simulink model "Electrical_System_2018b_obfs"  (R2019b)
settings: Solver=VariableStepAuto  StartTime=0.0  StopTime=5  RelTol=1e-3  AbsTol=1e-3  EnableMultiTasking=on
InitFcn:
  | Steady_State_Initialisation;
StopFcn:
  | %sscexplore(simlog);
  | %Logging
undefined symbols (not defined in the file): abrlhklxvp, aexgmhuedq, afmfmjnutg, afpphrjpnc, ahuxbyvruc, alarvljztt, amxnyqmnuw, aodrlwvqie, aolhmuplyq, aqpmguuqkg, auesgwirzl, aurophlnng, awamelrhru, ayfhvxflxn, azxkacuhqc, babszerikg, bawhdqanwq, bevoqecvei, bltjvqbchx, bmqsuewujl, bsmyqjfgnf, btvjbsmnve, bywgxqeadw, bziaduxaer, bzmcmdqocb, bzsvyvetat, ccsjnrbsih, cdvenygxwh, cedkrnslhx, cjheorclzs, cjrdshrtqx, ckhavyhcza, ckxewznhlz, cmrcgyiplk, conenicnws, cqkejbgjnn, csfnuwymhe, cunupkhwbh, cwzfvzuxxh, dcadmadufn, dcfponivnv, ddtrqjrhjn, dfhoxvkqas, dfrhtcwpne, dfvomcagjv, djijwylxea, dnmeqksrrm, dnzewbdkaa, dsqcykyxav, dtswwlttmm, ecumpidjtv, edegaywrct, ejjjsmnejc, eknqnehjdz, emvdetzouf, esxbqkbahr, etnkkbreiq, eunoiiiirw, ewewcuedir, fatkfxdhtc ... (+386)
libraries: fl_lib x802, ee_lib x362, fl_ps_legacy_lib x160, nesl_utility x85
(part 16 of 26)

== system Electrical_System_2018b_obfs/Redacted_1221/Redacted_7996/Redacted_2/Redacted_38/Redacted_8107/Redacted_7529 ==
  Redacted_1084 : ee_lib/Semiconductors & Converters/Diode  ModelType=izdobyzqle  Vf=evihkhstbw V  Ron=vuuzcskhxp Ohm  Goff=mlnvudefzh S  prmExp=lejtfyvyux  I12=tabfzyvjjw A  V12=fmhjbmpmqb V  IS=owmyvxeefr A  ec=svhshwyrgx  I1=ljwwgiysfr A  V1=cxpndjgyrh V  RS=xmnymghsco Ohm  Tmeas=zghhcluqyd degC  N_series=cpqweisfkm  N_parallel=lexvmnvtgk  Rz=qmwaibykde Ohm  BV=drbkvafvno V  C_param=xxddurxsbn  CJ=xdxqdbopkt pF  CJ0=kptwwgjzso pF  VJ=hkmlapdavl V  Mgrad=vyzsmtybaj  Vvec=idvcnbeqxi V  Cvec=lhhotedrtn pF  FC=bewrjixdsy  Q_param=ivgezzsvid  iRM=kttgtaurdl A  iF=feyuhnjntw A  didt=wzaronjtgo A/us  trr_factor=xjeyfathbr  trr=gmgemqpikq ns  Qrr=psqfrowxwi s*uA  TT=klclxejlrf ns  tau=dytmmyuhbl ns  T_param=gahisfowsc  IS_T2=cvrsutiwlp A  I1_T2=lhcryknhzp A  V1_T2=nabkspnaxp V  Tmeas2=yxgzayqlzi degC  EG_param=qwryskkgkm  EG=oxgfzaipim eV  XTI_param=bjoagcqjsw  XTI=ycmlwmcwwf  dBVdT=dotvxllash V/K  Tdevice=ezkzuymnag degC  i_specify=off  i_priority=None  i=daydkonpxs A  i_nominal_specify=off  i_nominal_unit=A  i_nominal_value=blmtdukctw  v_specify=off  v_priority=None  v=akgpvqsdrg V  v_nominal_specify=off  v_nominal_unit=V  v_nominal_value=lygvltjuxz  i_capacitor_specify=off  i_capacitor_priority=None  i_capacitor=btazvuzoqw A  i_capacitor_nominal_specify=off  i_capacitor_nominal_unit=A  i_capacitor_nominal_value=mpfscvienm  v_capacitor_specify=off  v_capacitor_priority=None  v_capacitor=fmmkhztbpm V  v_capacitor_nominal_specify=off  v_capacitor_nominal_unit=V  v_capacitor_nominal_value=ltvznzjvwn  power_dissipated_specify=off  power_dissipated_priority=None  power_dissipated=jxwbertlfp W  power_dissipated_nominal_specify=off  power_dissipated_nominal_unit=W  power_dissipated_nominal_value=qtoemtvmie  thermal_network_parameterization=vtcsjudzim  Rth=heeowetwuv K/W  Rth_Foster=ruqyjqugrl K/W  thermal_mass_parameterization=envbmlquin  thermal_mass=kwknucpqzf J/K  thermal_mass_Foster=cqdqbkuljl J/K  thermal_time_constant=ngzwrugeai s  thermal_time_constant_Foster=bpqkuoqgpu s  thermal_mass_initial_temperatures=rhqgsoeffv degC
      settings: SourceProductName=Simscape Electrical  InternalSimscapePortConfiguration="{\"Bottom\":[],\"Left\":[{\"id\":\"p\",\"label\":\"\",\"type\":\"foundation.electrical.electrical\"},{\"id\":\"H\",\"label\":\"H\",\"type\":\"foundation.thermal.thermal\"}],\"Right\":[{\"id\":\"n\",\"label\":\"\",\"type\":\"foundation.electrical.electrical\"}],\"Top\":[]}"
  Redacted_1116 : ee_lib/Semiconductors & Converters/Diode  ModelType=fezxkqjgqt  Vf=fxigmtorpi V  Ron=gczbijkgdb Ohm  Goff=eezdenrgyt S  prmExp=mooftzwsze  I12=hrjfyjjrls A  V12=rpjtpkqqat V  IS=wddelpkxcd A  ec=wnwrwrhrqv  I1=lxjmeqhfps A  V1=hwunywjuky V  RS=qeymtoopbm Ohm  Tmeas=moiijwwbbr degC  N_series=tpmlovrlqd  N_parallel=mfzinvasat  Rz=ovydxazbex Ohm  BV=pxxjbuwfqz V  C_param=qpcursofjw  CJ=xcjuvsuivt pF  CJ0=izhwoolfnz pF  VJ=vpiestyydi V  Mgrad=cktkfzulrn  Vvec=sciesnzgxa V  Cvec=ffirljqncp pF  FC=ggluskildl  Q_param=ivvyfxrgkf  iRM=vqdtwwvmky A  iF=pvrysfcrbt A  didt=aeuywekxid A/us  trr_factor=nqhyqwmkdj  trr=iqctnvzxva ns  Qrr=isykhlqcxv s*uA  TT=ebdjbikpxl ns  tau=braofdeijp ns  T_param=rwhudzydrl  IS_T2=ahyaxsqykv A  I1_T2=yqxbhliehb A  V1_T2=cahaepnczu V  Tmeas2=rcpxcpgkrc degC  EG_param=ajpcsxcgmn  EG=mkbrzouimp eV  XTI_param=fgrnhizmgq  XTI=rtivxbansn  dBVdT=bztvayfwko V/K  Tdevice=fwkbokttbz degC  i_specify=off  i_priority=None  i=frjerhxssh A  i_nominal_specify=off  i_nominal_unit=A  i_nominal_value=xtkoagasgf  v_specify=off  v_priority=None  v=ltequmallb V  v_nominal_specify=off  v_nominal_unit=V  v_nominal_value=nmmakwdacx  i_capacitor_specify=off  i_capacitor_priority=None  i_capacitor=oexcyamlgf A  i_capacitor_nominal_specify=off  i_capacitor_nominal_unit=A  i_capacitor_nominal_value=tsglkvwluo  v_capacitor_specify=off  v_capacitor_priority=None  v_capacitor=uttypvaate V  v_capacitor_nominal_specify=off  v_capacitor_nominal_unit=V  v_capacitor_nominal_value=rmuymllcxy  power_dissipated_specify=off  power_dissipated_priority=None  power_dissipated=pikztcggua W  power_dissipated_nominal_specify=off  power_dissipated_nominal_unit=W  power_dissipated_nominal_value=wdovbxesnv  thermal_network_parameterization=jzuiubyezr  Rth=zuswrtrzus K/W  Rth_Foster=mncqifigaw K/W  thermal_mass_parameterization=xdyzfyucfr  thermal_mass=digaqnegbt J/K  thermal_mass_Foster=rlibwejjxp J/K  thermal_time_constant=dtpvzfxfdr s  thermal_time_constant_Foster=lltkuepcfr s  thermal_mass_initial_temperatures=qrjsznixcz degC
      settings: SourceProductName=Simscape Electrical  InternalSimscapePortConfiguration="{\"Bottom\":[],\"Left\":[{\"id\":\"p\",\"label\":\"\",\"type\":\"foundation.electrical.electrical\"},{\"id\":\"H\",\"label\":\"H\",\"type\":\"foundation.thermal.thermal\"}],\"Right\":[{\"id\":\"n\",\"label\":\"\",\"type\":\"foundation.electrical.electrical\"}],\"Top\":[]}"
  Redacted_3535 : ee_lib/Passive/Thermal/Thermal Resistor  R=nnovauibfc K/W  T_specify=off  T_priority=None  T=smooypmoft K  T_nominal_specify=off  T_nominal_unit=K  T_nominal_value=kuntnrwjbm  Q_specify=off  Q_priority=None  Q=ffwudhgepl W  Q_nominal_specify=off  Q_nominal_unit=W  Q_nominal_value=dtpumxdoon
      settings: SourceProductName=Simscape Electrical  SourceProductBaseCode=PS  InternalSimscapePortConfiguration="{\"Bottom\":[],\"Left\":[{\"id\":\"A\",\"label\":\"A\",\"type\":\"foundation.thermal.thermal\"}],\"Right\":[{\"id\":\"B\",\"label\":\"B\",\"type\":\"foundation.thermal.thermal\"}],\"Top\":[]}"
  Redacted_4646 : fl_lib/Electrical/Electrical Elements/Switch  R_closed=pqgaemrczs Ohm  G_open=ijstyudrez 1/Ohm  Threshold=xtptocpmir  i_specify=off  i_priority=None  i=ciwbetxiqp A  i_nominal_specify=off  i_nominal_unit=A  i_nominal_value=enaqgcdnlz  v_specify=off  v_priority=None  v=vzxbmtbrih V  v_nominal_specify=off  v_nominal_unit=V  v_nominal_value=wsynujvvrc
      settings: SourceProductName=Simscape
  Redacted_5773 : ee_lib/Passive/Thermal/Thermal Resistor  R=edegaywrct K/W  T_specify=off  T_priority=None  T=ckxewznhlz K  T_nominal_specify=off  T_nominal_unit=K  T_nominal_value=gkohcrexhh  Q_specify=off  Q_priority=None  Q=ubkoftignu W  Q_nominal_specify=off  Q_nominal_unit=W  Q_nominal_value=dmlagltzis
      settings: SourceProductName=Simscape Electrical  SourceProductBaseCode=PS  InternalSimscapePortConfiguration="{\"Bottom\":[],\"Left\":[{\"id\":\"A\",\"label\":\"A\",\"type\":\"foundation.thermal.thermal\"}],\"Right\":[{\"id\":\"B\",\"label\":\"B\",\"type\":\"foundation.thermal.thermal\"}],\"Top\":[]}"
  Redacted_6378 : fl_lib/Electrical/Electrical Elements/Switch  R_closed=whblxebmyo Ohm  G_open=pswlapjyse 1/Ohm  Threshold=pwweavvhgn  i_specify=off  i_priority=None  i=elbzoqtfyk A  i_nominal_specify=off  i_nominal_unit=A  i_nominal_value=sbenumnblt  v_specify=off  v_priority=None  v=vclonruutc V  v_nominal_specify=off  v_nominal_unit=V  v_nominal_value=xzmfluzccj
      settings: SourceProductName=Simscape
  Redacted_6493 : ee_lib/Semiconductors & Converters/Diode  ModelType=vttiaricbl  Vf=ogmshccous V  Ron=clhmvbtmpj Ohm  Goff=qlartobjid S  prmExp=yehkiyfwrf  I12=uxupgfdefd A  V12=fnuyckqxoq V  IS=gijoawrwfl A  ec=jacbxiiccp  I1=fgncvolvfb A  V1=onmmvewocq V  RS=otizmpmqay Ohm  Tmeas=kapmscogpw degC  N_series=qithjwaybs  N_parallel=gzsiinkylg  Rz=mycurxzcbk Ohm  BV=rewmblcdnc V  C_param=whbhsgwygj  CJ=vcfjucyupa pF  CJ0=xlhglqasyv pF  VJ=qosroxbxnj V  Mgrad=hkxiwvlmct  Vvec=oruqsfqddv V  Cvec=sashthzyhc pF  FC=xhlcguewdu  Q_param=ixrezpchhb  iRM=djiqriviqu A  iF=hegkfqrgrh A  didt=xbnqhutjlk A/us  trr_factor=dzlursyiar  trr=ecuaptzqel ns  Qrr=imqebfbhyx s*uA  TT=dymphevecl ns  tau=sblfgxlvjk ns  T_param=xyqfplnupv  IS_T2=uxlhlnzgja A  I1_T2=cyfpvxxmef A  V1_T2=dbwddhswgd V  Tmeas2=zlvkqtpnfx degC  EG_param=fcgsavfugx  EG=jbtqkskxko eV  XTI_param=buvkrschfc  XTI=qctkrmjsmi  dBVdT=kyilrmqoag V/K  Tdevice=tvzbjueohw degC  i_specify=off  i_priority=None  i=wgxzavfjwv A  i_nominal_specify=off  i_nominal_unit=A  i_nominal_value=zeyksugkif  v_specify=off  v_priority=None  v=knzxvrfofm V  v_nominal_specify=off  v_nominal_unit=V  v_nominal_value=chjlmmweiu  i_capacitor_specify=off  i_capacitor_priority=None  i_capacitor=mednscufnd A  i_capacitor_nominal_specify=off  i_capacitor_nominal_unit=A  i_capacitor_nominal_value=leufklsnbm  v_capacitor_specify=off  v_capacitor_priority=None  v_capacitor=xrcvmsmjec V  v_capacitor_nominal_specify=off  v_capacitor_nominal_unit=V  v_capacitor_nominal_value=tbidastozp  power_dissipated_specify=off  power_dissipated_priority=None  power_dissipated=hpegcrwzwe W  power_dissipated_nominal_specify=off  power_dissipated_nominal_unit=W  power_dissipated_nominal_value=ueblnqxpvf  thermal_network_parameterization=hkgyvucefr  Rth=bprjyiudmm K/W  Rth_Foster=bqwxkgbgel K/W  thermal_mass_parameterization=gnzfaualyz  thermal_mass=qgoqgvzmhv J/K  thermal_mass_Foster=lrajjjlskm J/K  thermal_time_constant=ffhhmbgnyr s  thermal_time_constant_Foster=dwjhaccnar s  thermal_mass_initial_temperatures=clzednejpb degC
      settings: SourceProductName=Simscape Electrical  InternalSimscapePortConfiguration="{\"Bottom\":[],\"Left\":[{\"id\":\"p\",\"label\":\"\",\"type\":\"foundation.electrical.electrical\"},{\"id\":\"H\",\"label\":\"H\",\"type\":\"foundation.thermal.thermal\"}],\"Right\":[{\"id\":\"n\",\"label\":\"\",\"type\":\"foundation.electrical.electrical\"}],\"Top\":[]}"
  Redacted_6995 : ee_lib/Semiconductors & Converters/Diode  ModelType=jutammamgf  Vf=phixztrybu V  Ron=wnueokvcjp Ohm  Goff=tlbagzjnli S  prmExp=qepetuupwd  I12=pipfumlpkp A  V12=cvdomcruuy V  IS=caphgfqgul A  ec=bfsyyglqre  I1=chsqwrduxs A  V1=pnvjrtaaxm V  RS=lnonjcbaes Ohm  Tmeas=uqgbdgyiqe degC  N_series=wzcnpegdoc  N_parallel=vzpnmjfana  Rz=jvagvrqcvr Ohm  BV=iowbeuhkbn V  C_param=zuyiiufywv  CJ=iafdabsqml pF  CJ0=krrwskzkzk pF  VJ=hcozynotnd V  Mgrad=qgebppotct  Vvec=rsjrazbslf V  Cvec=tqthplanse pF  FC=ggxesrxcvy  Q_param=npdtukbqqy  iRM=baufngyjqn A  iF=eaqdcbooap A  didt=zpmwgjwvhg A/us  trr_factor=lxzhpepuka  trr=lxionuhlzp ns  Qrr=cedutijpwi s*uA  TT=unwcmeqxzu ns  tau=bqcttgeatr ns  T_param=hnuznnjugk  IS_T2=heqzetlzuz A  I1_T2=zuzqagssvf A  V1_T2=jebzqvibaa V  Tmeas2=liqnbtkzkz degC  EG_param=paovebrsxo  EG=afafawlgir eV  XTI_param=eznhhwiwyq  XTI=pnvwrinkhd  dBVdT=ncvzhuvhdd V/K  Tdevice=xjszywknrp degC  i_specify=off  i_priority=None  i=ksmvescqii A  i_nominal_specify=off  i_nominal_unit=A  i_nominal_value=vdbtoezmns  v_specify=off  v_priority=None  v=mjrlqidlhj V  v_nominal_specify=off  v_nominal_unit=V  v_nominal_value=kpyhvjeelx  i_capacitor_specify=off  i_capacitor_priority=None  i_capacitor=rleowstiyj A  i_capacitor_nominal_specify=off  i_capacitor_nominal_unit=A  i_capacitor_nominal_value=cqjcqxpbep  v_capacitor_specify=off  v_capacitor_priority=None  v_capacitor=atjaslazmh V  v_capacitor_nominal_specify=off  v_capacitor_nominal_unit=V  v_capacitor_nominal_value=wpxewlzklj  power_dissipated_specify=off  power_dissipated_priority=None  power_dissipated=mwdylpnyws W  power_dissipated_nominal_specify=off  power_dissipated_nominal_unit=W  power_dissipated_nominal_value=jrnlbozeni  thermal_network_parameterization=dbphpnpgiy  Rth=xxmcnnlxls K/W  Rth_Foster=owybowsyqi K/W  thermal_mass_parameterization=fipqtfbsom  thermal_mass=sufocoiqer J/K  thermal_mass_Foster=kpdllifdhl J/K  thermal_time_constant=miladgbser s  thermal_time_constant_Foster=ttjplmfpfh s  thermal_mass_initial_temperatures=yzetsrudhm degC
      settings: SourceProductName=Simscape Electrical  InternalSimscapePortConfiguration="{\"Bottom\":[],\"Left\":[{\"id\":\"p\",\"label\":\"\",\"type\":\"foundation.electrical.electrical\"},{\"id\":\"H\",\"label\":\"H\",\"type\":\"foundation.thermal.thermal\"}],\"Right\":[{\"id\":\"n\",\"label\":\"\",\"type\":\"foundation.electrical.electrical\"}],\"Top\":[]}"
  Redacted_7501 : fl_lib/Electrical/Electrical Elements/Switch  R_closed=hkpufaysry Ohm  G_open=gpzouyuqvs 1/Ohm  Threshold=qzaeawbkdg  i_specify=off  i_priority=None  i=gtsknxhqqy A  i_nominal_specify=off  i_nominal_unit=A  i_nominal_value=zlbtgeochj  v_specify=off  v_priority=None  v=dywgqxyfrf V  v_nominal_specify=off  v_nominal_unit=V  v_nominal_value=tmhxabklck
      settings: SourceProductName=Simscape
  Redacted_7912 : ee_lib/Semiconductors & Converters/Diode  ModelType=rwagzwdqyn  Vf=iprlzxekyz V  Ron=ezbutranua Ohm  Goff=dhqmfjsjtj S  prmExp=cuexlqtxbd  I12=huvborskst A  V12=yjowgrbbok V  IS=recqqdaika A  ec=maqoiaeowd  I1=dfgsziufhg A  V1=jfgkxmlxal V  RS=rwxzegglbh Ohm  Tmeas=jioffbrnci degC  N_series=fvxphqozbm  N_parallel=klvniviixg  Rz=lchiewuqih Ohm  BV=jvermwbkfz V  C_param=aeaujmzfqy  CJ=rqoxxznype pF  CJ0=fgmgeudhfq pF  VJ=dirbounqek V  Mgrad=rzoyersdzn  Vvec=uohghsdlzr V  Cvec=sbaqfspfgh pF  FC=nnbelozaaf  Q_param=otgxpunumz  iRM=nvsewfidxu A  iF=stbhkngzcy A  didt=qcdzydoljm A/us  trr_factor=finkzecfng  trr=obgbvrcfxj ns  Qrr=hjehgagare s*uA  TT=fxfsjglodu ns  tau=lgetnnmyzx ns  T_param=mpmzudimoq  IS_T2=ixsjntuwes A  I1_T2=nlkfhnvcta A  V1_T2=ihjdtzpuop V  Tmeas2=tlrwraxkbp degC  EG_param=xxzzjsgowy  EG=osmqxpygwj eV  XTI_param=xnphfrlzyj  XTI=lyfutvjcve  dBVdT=zpjxgnsdoi V/K  Tdevice=ejwhigvruq degC  i_specify=off  i_priority=None  i=fjexkzazrq A  i_nominal_specify=off  i_nominal_unit=A  i_nominal_value=fuktovoelv  v_specify=off  v_priority=None  v=wqxfyskvyj V  v_nominal_specify=off  v_nominal_unit=V  v_nominal_value=kqzybxpjnu  i_capacitor_specify=off  i_capacitor_priority=None  i_capacitor=ofanbrxoer A  i_capacitor_nominal_specify=off  i_capacitor_nominal_unit=A  i_capacitor_nominal_value=joivzqgqdu  v_capacitor_specify=off  v_capacitor_priority=None  v_capacitor=slkzwjrqcn V  v_capacitor_nominal_specify=off  v_capacitor_nominal_unit=V  v_capacitor_nominal_value=btklwtqjaq  power_dissipated_specify=off  power_dissipated_priority=None  power_dissipated=bkyjzqujvp W  power_dissipated_nominal_specify=off  power_dissipated_nominal_unit=W  power_dissipated_nominal_value=wvaevrhbzy  thermal_network_parameterization=ntnnypyupt  Rth=fjtewgrqlr K/W  Rth_Foster=rcjajmoogt K/W  thermal_mass_parameterization=wipcxjewms  thermal_mass=ljwuxclnun J/K  thermal_mass_Foster=llxyimdsaa J/K  thermal_time_constant=dxqpwebpua s  thermal_time_constant_Foster=pglxwtomtd s  thermal_mass_initial_temperatures=hidbrzofoy degC
      settings: SourceProductName=Simscape Electrical  InternalSimscapePortConfiguration="{\"Bottom\":[],\"Left\":[{\"id\":\"p\",\"label\":\"\",\"type\":\"foundation.electrical.electrical\"},{\"id\":\"H\",\"label\":\"H\",\"type\":\"foundation.thermal.thermal\"}],\"Right\":[{\"id\":\"n\",\"label\":\"\",\"type\":\"foundation.electrical.electrical\"}],\"Top\":[]}"
  Redacted_8948 : ee_lib/Semiconductors & Converters/Diode  ModelType=zkbpdzndof  Vf=kzhddisigf V  Ron=dwbhxmmusu Ohm  Goff=bovrirpbke S  prmExp=ivxatfylqk  I12=zvwbuodsjc A  V12=hygnuemoix V  IS=tfwnmkcsyy A  ec=zckyboqwbh  I1=gvubnhdebg A  V1=kunekwhnwv V  RS=ecflormmke Ohm  Tmeas=gtkqfbhchd degC  N_series=zexkrzwhec  N_parallel=wsgrspekur  Rz=shpvzfgjkm Ohm  BV=ccrgfqifiu V  C_param=jqwkikvznj  CJ=pnytyzyvdj pF  CJ0=lnkqhrgppk pF  VJ=uipwhuhyam V  Mgrad=iufkrvrvhb  Vvec=xkhpmfjhdd V  Cvec=uybicdtekz pF  FC=fimwjtluum  Q_param=ctngtcsbuv  iRM=irhzfxednb A  iF=qottmbjvjb A  didt=eltqzqpenk A/us  trr_factor=vqicmosdaw  trr=wqdiphslkd ns  Qrr=xasjjvxkjf s*uA  TT=lfeufmusqp ns  tau=blqvezoiur ns  T_param=okzhatcrhj  IS_T2=cdpladztvs A  I1_T2=cfzfnsrxin A  V1_T2=isvyuxqhap V  Tmeas2=uhkmdahdaa degC  EG_param=hrwywwihcq  EG=euxrsrmpjb eV  XTI_param=yykzdnakfo  XTI=zqzfakywur  dBVdT=yajojhgtsn V/K  Tdevice=hzqpbccwul degC  i_specify=off  i_priority=None  i=nyprrbxiwt A  i_nominal_specify=off  i_nominal_unit=A  i_nominal_value=qchgoadyeu  v_specify=off  v_priority=None  v=cxjaxlbuuh V  v_nominal_specify=off  v_nominal_unit=V  v_nominal_value=enugljpiad  i_capacitor_specify=off  i_capacitor_priority=None  i_capacitor=fyumucjymc A  i_capacitor_nominal_specify=off  i_capacitor_nominal_unit=A  i_capacitor_nominal_value=mwslhozglg  v_capacitor_specify=off  v_capacitor_priority=None  v_capacitor=hatozsragm V  v_capacitor_nominal_specify=off  v_capacitor_nominal_unit=V  v_capacitor_nominal_value=nedivgajsa  power_dissipated_specify=off  power_dissipated_priority=None  power_dissipated=dxpmizpfad W  power_dissipated_nominal_specify=off  power_dissipated_nominal_unit=W  power_dissipated_nominal_value=mfhacyeutq  thermal_network_parameterization=kkiafvbnuz  Rth=dhbknzzzyf K/W  Rth_Foster=krirsjbigm K/W  thermal_mass_parameterization=ncxhbuwddl  thermal_mass=ixwloffvbv J/K  thermal_mass_Foster=ysigxentbo J/K  thermal_time_constant=xcztavzciz s  thermal_time_constant_Foster=ysamghlcvt s  thermal_mass_initial_temperatures=bozfzmyjvc degC
      settings: SourceProductName=Simscape Electrical  InternalSimscapePortConfiguration="{\"Bottom\":[],\"Left\":[{\"id\":\"p\",\"label\":\"\",\"type\":\"foundation.electrical.electrical\"},{\"id\":\"H\",\"label\":\"H\",\"type\":\"foundation.thermal.thermal\"}],\"Right\":[{\"id\":\"n\",\"label\":\"\",\"type\":\"foundation.electrical.electrical\"}],\"Top\":[]}"
  Redacted_9145 : ee_lib/Passive/Thermal/Thermal Resistor  R=ayfhvxflxn K/W  T_specify=off  T_priority=None  T=tjccnrtnkd K  T_nominal_specify=off  T_nominal_unit=K  T_nominal_value=fepcbhdcxp  Q_specify=off  Q_priority=None  Q=yjxepqleci W  Q_nominal_specify=off  Q_nominal_unit=W  Q_nominal_value=ednxibyxiq
      settings: SourceProductName=Simscape Electrical  SourceProductBaseCode=PS  InternalSimscapePortConfiguration="{\"Bottom\":[],\"Left\":[{\"id\":\"A\",\"label\":\"A\",\"type\":\"foundation.thermal.thermal\"}],\"Right\":[{\"id\":\"B\",\"label\":\"B\",\"type\":\"foundation.thermal.thermal\"}],\"Top\":[]}"
  Redacted_9512 : ee_lib/Passive/Thermal/Thermal Resistor  R=qdhdwuufms K/W  T_specify=off  T_priority=None  T=qpsjblfwaq K  T_nominal_specify=off  T_nominal_unit=K  T_nominal_value=jijbdnsmls  Q_specify=off  Q_priority=None  Q=isaanbfiuu W  Q_nominal_specify=off  Q_nominal_unit=W  Q_nominal_value=pquhzcjzlx
      settings: SourceProductName=Simscape Electrical  SourceProductBaseCode=PS  InternalSimscapePortConfiguration="{\"Bottom\":[],\"Left\":[{\"id\":\"A\",\"label\":\"A\",\"type\":\"foundation.thermal.thermal\"}],\"Right\":[{\"id\":\"B\",\"label\":\"B\",\"type\":\"foundation.thermal.thermal\"}],\"Top\":[]}"
  Redacted_3998 : PMIOPort  Side=Left
  Redacted_3025 : PMIOPort  Port=2  Side=Left
  Redacted_376 : PMIOPort  Port=3  Side=Left
  Redacted_4990 : PMIOPort  Port=4  Side=Right
  Redacted_668 : PMIOPort  Port=5  Side=Right
  Redacted_6324 : PMIOPort  Port=6  Side=Right
  Redacted_5539 : PMIOPort  Port=7  Side=Left
  Redacted_7776 : PMIOPort  Port=8  Side=Right
  connections:
  Redacted_6493/LConn1 -- Redacted_3025/RConn1 -- Redacted_1116/RConn1
  Redacted_6493/RConn1 -- Redacted_4646/LConn1 -- Redacted_1116/LConn1
  Redacted_5773/LConn1 -- Redacted_8948/LConn2 -- Redacted_1084/LConn2
  Redacted_4990/RConn1 -- Redacted_6378/RConn2
  Redacted_1084/LConn1 -- Redacted_6378/LConn1 -- Redacted_8948/RConn1
  Redacted_8948/LConn1 -- Redacted_3998/RConn1 -- Redacted_1084/RConn1
  Redacted_9145/RConn1 -- Redacted_3535/RConn1 -- Redacted_9512/LConn1 -- Redacted_5773/RConn1
  Redacted_7912/LConn1 -- Redacted_376/RConn1 -- Redacted_6995/RConn1
  Redacted_6324/RConn1 -- Redacted_7501/RConn2
  Redacted_7776/RConn1 -- Redacted_7501/RConn1 -- Redacted_4646/RConn1 -- Redacted_6378/RConn1
  Redacted_668/RConn1 -- Redacted_4646/RConn2
  Redacted_6995/LConn1 -- Redacted_7501/LConn1 -- Redacted_7912/RConn1
  Redacted_6995/LConn2 -- Redacted_3535/LConn1 -- Redacted_7912/LConn2
  Redacted_9512/RConn1 -- Redacted_5539/RConn1
  Redacted_6493/LConn2 -- Redacted_1116/LConn2 -- Redacted_9145/LConn1

== system Electrical_System_2018b_obfs/Redacted_1221/Redacted_7996/Redacted_2/Redacted_38/Redacted_8107/Redacted_8444 ==
  Neutral_Negative : Subsystem  VariantControl=Variant1
  Positive_Neutral : Subsystem  VariantControl=Variant3
  Redacted_3917 : Subsystem  VariantControl=Variant2
  Redacted_8974 : PMIOPort  Side=Left
  Redacted_9727 : PMIOPort  Port=2  Side=Left
  Redacted_5818 : PMIOPort  Port=3  Side=Left
  Redacted_9930 : PMIOPort  Port=4  Side=Right
  Redacted_8840 : PMIOPort  Port=5  Side=Right

== system Electrical_System_2018b_obfs/Redacted_1221/Redacted_7996/Redacted_7418/Redacted_4377/Redacted_6082/Redacted_1335 ==
  Redacted_1591 : ee_lib/Semiconductors & Converters/Diode  ModelType=eepsypmlnm  Vf=vsdkpxkdvt V  Ron=hvipwyltcs Ohm  Goff=pncgtdpcky S  prmExp=ywnmgnebdg  I12=pijcksfllq A  V12=sokkewuwnq V  IS=lenjbmkbmu A  ec=usrydsfczj  I1=diflzejvue A  V1=ondqlqjixt V  RS=mmlszzuage Ohm  Tmeas=npymjxtxff degC  N_series=uwgycohtvj  N_parallel=vvktvyaksv  Rz=csndwjwvcs Ohm  BV=siuhniwsas V  C_param=mqmeyzacus  CJ=pspkjiflhw pF  CJ0=mkzhvuscrv pF  VJ=cxyxmemllb V  Mgrad=kwjdstgiqi  Vvec=rfkmbedwbl V  Cvec=tzcpccccyr pF  FC=tzhyramxnn  Q_param=jtaiadwcvb  iRM=teewqjimfa A  iF=dkuaowzmzk A  didt=wswqfekgti A/us  trr_factor=vgbmpjncqd  trr=qytitrwxvl ns  Qrr=jukjiwceed s*uA  TT=vfhkswzpii ns  tau=bcxefnpqla ns  T_param=knzoykoruc  IS_T2=wmrtfwgfyn A  I1_T2=wwatewxxmj A  V1_T2=vcmdipevcj V  Tmeas2=slejovgnym degC  EG_param=yrmdwgjpga  EG=obqdoxighd eV  XTI_param=hiiulsmtnp  XTI=fzvxbjgrlx  dBVdT=tcetjpxzuo V/K  Tdevice=jhymtvpuuv degC  i_specify=off  i_priority=None  i=lxkrvrufkt A  i_nominal_specify=off  i_nominal_unit=A  i_nominal_value=fptpkrapsh  v_specify=off  v_priority=None  v=hnwpggrdrb V  v_nominal_specify=off  v_nominal_unit=V  v_nominal_value=loyliznani  i_capacitor_specify=off  i_capacitor_priority=None  i_capacitor=qntetqcfew A  i_capacitor_nominal_specify=off  i_capacitor_nominal_unit=A  i_capacitor_nominal_value=bhetqfpmna  v_capacitor_specify=off  v_capacitor_priority=None  v_capacitor=qmuuchuxyz V  v_capacitor_nominal_specify=off  v_capacitor_nominal_unit=V  v_capacitor_nominal_value=vvvpkitexs  power_dissipated_specify=off  power_dissipated_priority=None  power_dissipated=kbjvtlpgfd W  power_dissipated_nominal_specify=off  power_dissipated_nominal_unit=W  power_dissipated_nominal_value=jvdnwocntn  thermal_network_parameterization=yoawbybtkl  Rth=uknyprueob K/W  Rth_Foster=quhjgsiudl K/W  thermal_mass_parameterization=atrvywscev  thermal_mass=gtmjoozywy J/K  thermal_mass_Foster=hdtqidrsds J/K  thermal_time_constant=adrtjfdoqm s  thermal_time_constant_Foster=lcosfsblai s  thermal_mass_initial_temperatures=kqftjagahg degC
      settings: SourceProductName=Simscape Electrical  InternalSimscapePortConfiguration="{\"Bottom\":[],\"Left\":[{\"id\":\"p\",\"label\":\"\",\"type\":\"foundation.electrical.electrical\"},{\"id\":\"H\",\"label\":\"H\",\"type\":\"foundation.thermal.thermal\"}],\"Right\":[{\"id\":\"n\",\"label\":\"\",\"type\":\"foundation.electrical.electrical\"}],\"Top\":[]}"
  Redacted_1669 : ee_lib/Passive/Thermal/Thermal Resistor  R=ejjjsmnejc K/W  T_specify=off  T_priority=None  T=mbytgkvqdk K  T_nominal_specify=off  T_nominal_unit=K  T_nominal_value=uvrqbhbcsu  Q_specify=off  Q_priority=None  Q=fryoumgfor W  Q_nominal_specify=off  Q_nominal_unit=W  Q_nominal_value=qudqfymccr
      settings: SourceProductName=Simscape Electrical  SourceProductBaseCode=PS  InternalSimscapePortConfiguration="{\"Bottom\":[],\"Left\":[{\"id\":\"A\",\"label\":\"A\",\"type\":\"foundation.thermal.thermal\"}],\"Right\":[{\"id\":\"B\",\"label\":\"B\",\"type\":\"foundation.thermal.thermal\"}],\"Top\":[]}"
  Redacted_4093 : fl_lib/Electrical/Electrical Elements/Switch  R_closed=bbadzxwyew Ohm  G_open=fzmtkxgwpd 1/Ohm  Threshold=dfvomcagjv  i_specify=off  i_priority=None  i=ohbeugqvip A  i_nominal_specify=off  i_nominal_unit=A  i_nominal_value=exxqjlbakz  v_specify=off  v_priority=None  v=rdiaxwucpj V  v_nominal_specify=off  v_nominal_unit=V  v_nominal_value=azkctcjsnz
      settings: SourceProductName=Simscape
  Redacted_5466 : ee_lib/Passive/Thermal/Thermal Resistor  R=wdtmondimm K/W  T_specify=off  T_priority=None  T=wrtafdzvbh K  T_nominal_specify=off  T_nominal_unit=K  T_nominal_value=fiihiabjan  Q_specify=off  Q_priority=None  Q=ypouestzei W  Q_nominal_specify=off  Q_nominal_unit=W  Q_nominal_value=mabqlhycjh
      settings: SourceProductName=Simscape Electrical  SourceProductBaseCode=PS  InternalSimscapePortConfiguration="{\"Bottom\":[],\"Left\":[{\"id\":\"A\",\"label\":\"A\",\"type\":\"foundation.thermal.thermal\"}],\"Right\":[{\"id\":\"B\",\"label\":\"B\",\"type\":\"foundation.thermal.thermal\"}],\"Top\":[]}"
  Redacted_7324 : fl_lib/Electrical/Electrical Elements/Switch  R_closed=omfvajnpfd Ohm  G_open=ipqnezpryn 1/Ohm  Threshold=mmcsavdyob  i_specify=off  i_priority=None  i=qwnjhvyruv A  i_nominal_specify=off  i_nominal_unit=A  i_nominal_value=zmauchnwye  v_specify=off  v_priority=None  v=ufnknxdamw V  v_nominal_specify=off  v_nominal_unit=V  v_nominal_value=edufhutzre
      settings: SourceProductName=Simscape
  Redacted_9050 : ee_lib/Passive/Thermal/Thermal Resistor  R=gnxjfqgycd K/W  T_specify=off  T_priority=None  T=dtswwlttmm K  T_nominal_specify=off  T_nominal_unit=K  T_nominal_value=iuxynuhpbk  Q_specify=off  Q_priority=None  Q=etqvxuddqu W  Q_nominal_specify=off  Q_nominal_unit=W  Q_nominal_value=jpdxcuslyz
      settings: SourceProductName=Simscape Electrical  SourceProductBaseCode=PS  InternalSimscapePortConfiguration="{\"Bottom\":[],\"Left\":[{\"id\":\"A\",\"label\":\"A\",\"type\":\"foundation.thermal.thermal\"}],\"Right\":[{\"id\":\"B\",\"label\":\"B\",\"type\":\"foundation.thermal.thermal\"}],\"Top\":[]}"
  Redacted_998 : ee_lib/Semiconductors & Converters/Diode  ModelType=jjfughauiv  Vf=eaqvjmxxyg V  Ron=canwxvkyyq Ohm  Goff=fylhafqfdf S  prmExp=dyvujabdmn  I12=kttaerjvea A  V12=kesibchmqe V  IS=cnmgoowrsx A  ec=wmgmtbxlpj  I1=kbcmpxrtrl A  V1=bxdgeigcbm V  RS=aqtkcecpuq Ohm  Tmeas=jagkxxxouu degC  N_series=eijeaxwsbs  N_parallel=gnezyptovg  Rz=ccfbjkqckh Ohm  BV=ibaqbmeitx V  C_param=qbielwnwyc  CJ=zriiuwgwxe pF  CJ0=dfescxdcew pF  VJ=cbwvhwuxfk V  Mgrad=imxnoqiriq  Vvec=scyvszjglj V  Cvec=fxqxkbblsd pF  FC=oefuhmbbrj  Q_param=azpytwrwfh  iRM=vffiognxml A  iF=obozmuzsag A  didt=gxjsoognzt A/us  trr_factor=ngilewgegt  trr=udeiywtgjk ns  Qrr=lseeyedphz s*uA  TT=rsgjgrebyr ns  tau=fnsxhspmvy ns  T_param=ompevgbwln  IS_T2=czoaxjmnms A  I1_T2=fomygjynsp A  V1_T2=axnvwvykbq V  Tmeas2=acusxjthih degC  EG_param=jvdcorncji  EG=cjbueeqdfy eV  XTI_param=ksyxmxcrgv  XTI=lqwkbkflhk  dBVdT=gzrvmvfdkg V/K  Tdevice=btlrowuowx degC  i_specify=off  i_priority=None  i=cbrwwtdksz A  i_nominal_specify=off  i_nominal_unit=A  i_nominal_value=tdaqsczgka  v_specify=off  v_priority=None  v=hzgsyifftd V  v_nominal_specify=off  v_nominal_unit=V  v_nominal_value=wwgtgaavtg  i_capacitor_specify=off  i_capacitor_priority=None  i_capacitor=ghdwybcfnr A  i_capacitor_nominal_specify=off  i_capacitor_nominal_unit=A  i_capacitor_nominal_value=patoccuvbb  v_capacitor_specify=off  v_capacitor_priority=None  v_capacitor=kipgljoorb V  v_capacitor_nominal_specify=off  v_capacitor_nominal_unit=V  v_capacitor_nominal_value=dyvrmzctdc  power_dissipated_specify=off  power_dissipated_priority=None  power_dissipated=ttfhebcktj W  power_dissipated_nominal_specify=off  power_dissipated_nominal_unit=W  power_dissipated_nominal_value=repcdnmkvu  thermal_network_parameterization=fmvbkiqdne  Rth=pazmfgafaa K/W  Rth_Foster=brspocefdd K/W  thermal_mass_parameterization=ykylewhfcq  thermal_mass=lrrjyxxvqd J/K  thermal_mass_Foster=vdbqyqwkrw J/K  thermal_time_constant=exusymqbix s  thermal_time_constant_Foster=asebieqyaj s  thermal_mass_initial_temperatures=hpkeovjooi degC
      settings: SourceProductName=Simscape Electrical  InternalSimscapePortConfiguration="{\"Bottom\":[],\"Left\":[{\"id\":\"p\",\"label\":\"\",\"type\":\"foundation.electrical.electrical\"},{\"id\":\"H\",\"label\":\"H\",\"type\":\"foundation.thermal.thermal\"}],\"Right\":[{\"id\":\"n\",\"label\":\"\",\"type\":\"foundation.electrical.electrical\"}],\"Top\":[]}"
  Redacted_3665 : PMIOPort  Side=Left
  Redacted_9500 : PMIOPort  Port=2  Side=Left
  Redacted_4916 : PMIOPort  Port=3  Side=Right
  Redacted_8865 : PMIOPort  Port=4  Side=Right
  Redacted_5813 : PMIOPort  Port=5  Side=Left
  Redacted_175 : PMIOPort  Port=6  Side=Right
  connections:
  Redacted_998/LConn2 -- Redacted_5466/LConn1
  Redacted_9050/RConn1 -- Redacted_5813/RConn1
  Redacted_8865/RConn1 -- Redacted_7324/RConn2
  Redacted_4093/RConn1 -- Redacted_7324/RConn1 -- Redacted_175/RConn1
  Redacted_1669/RConn1 -- Redacted_9050/LConn1 -- Redacted_5466/RConn1
  Redacted_3665/RConn1 -- Redacted_1591/RConn1
  Redacted_1591/LConn1 -- Redacted_4093/LConn1
  Redacted_4916/RConn1 -- Redacted_4093/RConn2
  Redacted_1591/LConn2 -- Redacted_1669/LConn1
  Redacted_998/RConn1 -- Redacted_7324/LConn1
  Redacted_998/LConn1 -- Redacted_9500/RConn1

== system Electrical_System_2018b_obfs/Redacted_1221/Redacted_7996/Redacted_7418/Redacted_4377/Redacted_6082/Redacted_1337 ==
  Redacted_1292 : ee_lib/Passive/Thermal/Thermal Resistor  R=gfxbaoqbci K/W  T_specify=off  T_priority=None  T=rvwtgoykrz K  T_nominal_specify=off  T_nominal_unit=K  T_nominal_value=dmbpfjxefx  Q_specify=off  Q_priority=None  Q=ozjvrxmttl W  Q_nominal_specify=off  Q_nominal_unit=W  Q_nominal_value=utwlydmrkv
      settings: SourceProductName=Simscape Electrical  SourceProductBaseCode=PS  InternalSimscapePortConfiguration="{\"Bottom\":[],\"Left\":[{\"id\":\"A\",\"label\":\"A\",\"type\":\"foundation.thermal.thermal\"}],\"Right\":[{\"id\":\"B\",\"label\":\"B\",\"type\":\"foundation.thermal.thermal\"}],\"Top\":[]}"
  Redacted_2743 : fl_lib/Electrical/Electrical Elements/Switch  R_closed=fsyfpyiukg Ohm  G_open=tvcalsacmg 1/Ohm  Threshold=ttjzchmxti  i_specify=off  i_priority=None  i=alduyvsbin A  i_nominal_specify=off  i_nominal_unit=A  i_nominal_value=loyuiwztoz  v_specify=off  v_priority=None  v=yjwvqchbme V  v_nominal_specify=off  v_nominal_unit=V  v_nominal_value=gjoornamne
      settings: SourceProductName=Simscape
  Redacted_3949 : ee_lib/Passive/Thermal/Thermal Resistor  R=mlcqaguecq K/W  T_specify=off  T_priority=None  T=hfikrglmxq K  T_nominal_specify=off  T_nominal_unit=K  T_nominal_value=dqcyvveaih  Q_specify=off  Q_priority=None  Q=qlchfeptuj W  Q_nominal_specify=off  Q_nominal_unit=W  Q_nominal_value=wfdtozcpan
      settings: SourceProductName=Simscape Electrical  SourceProductBaseCode=PS  InternalSimscapePortConfiguration="{\"Bottom\":[],\"Left\":[{\"id\":\"A\",\"label\":\"A\",\"type\":\"foundation.thermal.thermal\"}],\"Right\":[{\"id\":\"B\",\"label\":\"B\",\"type\":\"foundation.thermal.thermal\"}],\"Top\":[]}"
  Redacted_4700 : ee_lib/Passive/Thermal/Thermal Resistor  R=gvbddagohg K/W  T_specify=off  T_priority=None  T=qxaoehcsep K  T_nominal_specify=off  T_nominal_unit=K  T_nominal_value=nuvljcivmd  Q_specify=off  Q_priority=None  Q=cuqzitalwz W  Q_nominal_specify=off  Q_nominal_unit=W  Q_nominal_value=fpqwunqvoe
      settings: SourceProductName=Simscape Electrical  SourceProductBaseCode=PS  InternalSimscapePortConfiguration="{\"Bottom\":[],\"Left\":[{\"id\":\"A\",\"label\":\"A\",\"type\":\"foundation.thermal.thermal\"}],\"Right\":[{\"id\":\"B\",\"label\":\"B\",\"type\":\"foundation.thermal.thermal\"}],\"Top\":[]}"
  Redacted_6636 : fl_lib/Electrical/Electrical Elements/Switch  R_closed=cxbeobdwcz Ohm  G_open=vivqqcjshk 1/Ohm  Threshold=ihvrcphyhk  i_specify=off  i_priority=None  i=tlqvhosmyx A  i_nominal_specify=off  i_nominal_unit=A  i_nominal_value=zlqewbizhg  v_specify=off  v_priority=None  v=bylehoytgr V  v_nominal_specify=off  v_nominal_unit=V  v_nominal_value=nrfabisoae
      settings: SourceProductName=Simscape
  Redacted_7671 : ee_lib/Semiconductors & Converters/Diode  ModelType=olgpyqkyap  Vf=yiidzvusor V  Ron=onikhigqex Ohm  Goff=zwvbfgfjia S  prmExp=mbejlzmzoi  I12=iqvhxxtdcy A  V12=plenerjsyz V  IS=seajxixdni A  ec=smzaoqkpfi  I1=srlrouujzp A  V1=pbinkrtesx V  RS=maerkwpvvt Ohm  Tmeas=boxaemfztm degC  N_series=zwoiykegtu  N_parallel=jpsnlhanqe  Rz=rbegpmpdpq Ohm  BV=xqcgehksui V  C_param=smmkeyjtrn  CJ=mxoawofixc pF  CJ0=ucwkumcrgx pF  VJ=flpomdjhqn V  Mgrad=pogzifmwhx  Vvec=lvysrprkky V  Cvec=ofowmtrtdp pF  FC=xzrncupysx  Q_param=dpijdlsbtg  iRM=imlwlhdaoz A  iF=zahcqmmmsp A  didt=srqymkpvtu A/us  trr_factor=qutyflkerp  trr=alnpfsdzft ns  Qrr=pnoodsbkqz s*uA  TT=qzjfylnffu ns  tau=fiwiuyhrdw ns  T_param=wjqxjtpsrv  IS_T2=gnlmqposwz A  I1_T2=hhxkfrkipw A  V1_T2=otwkxldrvh V  Tmeas2=pqzzkcslrw degC  EG_param=rgdwepjzgz  EG=towtzjxupc eV  XTI_param=wnrxgiphjy  XTI=ifqnzmcann  dBVdT=izcgyclarw V/K  Tdevice=kuguckrfas degC  i_specify=off  i_priority=None  i=qwraxdsfza A  i_nominal_specify=off  i_nominal_unit=A  i_nominal_value=jrebnsmptq  v_specify=off  v_priority=None  v=faivdficoh V  v_nominal_specify=off  v_nominal_unit=V  v_nominal_value=bfbyoqyboc  i_capacitor_specify=off  i_capacitor_priority=None  i_capacitor=jrptblagdq A  i_capacitor_nominal_specify=off  i_capacitor_nominal_unit=A  i_capacitor_nominal_value=nibfyfosby  v_capacitor_specify=off  v_capacitor_priority=None  v_capacitor=whspnfsgdn V  v_capacitor_nominal_specify=off  v_capacitor_nominal_unit=V  v_capacitor_nominal_value=edempxzddr  power_dissipated_specify=off  power_dissipated_priority=None  power_dissipated=peqvvccveb W  power_dissipated_nominal_specify=off  power_dissipated_nominal_unit=W  power_dissipated_nominal_value=fvdlfslssq  thermal_network_parameterization=svzrqymosw  Rth=pzdrjrnlgr K/W  Rth_Foster=acztezytnk K/W  thermal_mass_parameterization=rgscyvsrgf  thermal_mass=kygdzlscru J/K  thermal_mass_Foster=dvwwklbogc J/K  thermal_time_constant=ykfmdcuqty s  thermal_time_constant_Foster=wgtknjdmmg s  thermal_mass_initial_temperatures=gjuzcynxks degC
      settings: SourceProductName=Simscape Electrical  InternalSimscapePortConfiguration="{\"Bottom\":[],\"Left\":[{\"id\":\"p\",\"label\":\"\",\"type\":\"foundation.electrical.electrical\"},{\"id\":\"H\",\"label\":\"H\",\"type\":\"foundation.thermal.thermal\"}],\"Right\":[{\"id\":\"n\",\"label\":\"\",\"type\":\"foundation.electrical.electrical\"}],\"Top\":[]}"
  Redacted_7804 : ee_lib/Semiconductors & Converters/Diode  ModelType=semwhebdsx  Vf=wlzsjodvxe V  Ron=kjejwwsved Ohm  Goff=idmqtjqxyt S  prmExp=ybznmgfoim  I12=ypbwuazhvu A  V12=kqbjrekczm V  IS=hvghirmuer A  ec=szvhwtedho  I1=dgebikxuyu A  V1=ekmofvolqe V  RS=jkmhfachtm Ohm  Tmeas=ahwyvfcpsr degC  N_series=atodrtceph  N_parallel=fkaurojkbb  Rz=egfgmfcnxn Ohm  BV=nluxtwjaqz V  C_param=qwanuoxlyf  CJ=ezbprdeztn pF  CJ0=peskbsrzop pF  VJ=vquvaidumd V  Mgrad=dfrmgpetae  Vvec=gunyxlsjla V  Cvec=nljyfkzkue pF  FC=itkqjjkjyc  Q_param=jgelcbblhx  iRM=jgdtjqhets A  iF=owsoaymscw A  didt=qmpgbmxkte A/us  trr_factor=hklhqkgxog  trr=veyznjjddh ns  Qrr=ejjniorttw s*uA  TT=suevkibuvy ns  tau=mawzmcgeyp ns  T_param=vqrqwbsxyj  IS_T2=ssgvnzergm A  I1_T2=kvtrmiebrl A  V1_T2=wfzbyspvvb V  Tmeas2=oidirsmqgk degC  EG_param=zfeizsafro  EG=pynrradmvc eV  XTI_param=chffuchcuy  XTI=acqdodawvu  dBVdT=ocrbmtpnpr V/K  Tdevice=zuabybkowd degC  i_specify=off  i_priority=None  i=bcjxinvzmi A  i_nominal_specify=off  i_nominal_unit=A  i_nominal_value=ackfofeggx  v_specify=off  v_priority=None  v=nodroimedg V  v_nominal_specify=off  v_nominal_unit=V  v_nominal_value=nhpkywzxmk  i_capacitor_specify=off  i_capacitor_priority=None  i_capacitor=gbqfpnudcs A  i_capacitor_nominal_specify=off  i_capacitor_nominal_unit=A  i_capacitor_nominal_value=jfrtogbkdj  v_capacitor_specify=off  v_capacitor_priority=None  v_capacitor=kykdbedtbj V  v_capacitor_nominal_specify=off  v_capacitor_nominal_unit=V  v_capacitor_nominal_value=bwzkdbziru  power_dissipated_specify=off  power_dissipated_priority=None  power_dissipated=crijfdzbch W  power_dissipated_nominal_specify=off  power_dissipated_nominal_unit=W  power_dissipated_nominal_value=gueeagjtzs  thermal_network_parameterization=nshhtosrtp  Rth=ymvhergmsa K/W  Rth_Foster=loktjbqqnk K/W  thermal_mass_parameterization=nxtgvvflim  thermal_mass=ipqsjmpyeh J/K  thermal_mass_Foster=pnnymgjcyt J/K  thermal_time_constant=fqlitfupll s  thermal_time_constant_Foster=ouoyijytio s  thermal_mass_initial_temperatures=hosplxrwnn degC
      settings: SourceProductName=Simscape Electrical  InternalSimscapePortConfiguration="{\"Bottom\":[],\"Left\":[{\"id\":\"p\",\"label\":\"\",\"type\":\"foundation.electrical.electrical\"},{\"id\":\"H\",\"label\":\"H\",\"type\":\"foundation.thermal.thermal\"}],\"Right\":[{\"id\":\"n\",\"label\":\"\",\"type\":\"foundation.electrical.electrical\"}],\"Top\":[]}"
  Redacted_9723 : PMIOPort  Side=Left
  Redacted_1721 : PMIOPort  Port=2  Side=Left
  Redacted_9002 : PMIOPort  Port=3  Side=Right
  Redacted_1469 : PMIOPort  Port=4  Side=Right
  Redacted_6509 : PMIOPort  Port=5  Side=Left
  Redacted_1134 : PMIOPort  Port=6  Side=Right
  connections:
  Redacted_7671/LConn2 -- Redacted_3949/LConn1
  Redacted_4700/RConn1 -- Redacted_6509/RConn1
  Redacted_1469/RConn1 -- Redacted_6636/RConn2
  Redacted_2743/RConn1 -- Redacted_6636/RConn1 -- Redacted_1134/RConn1
  Redacted_1292/RConn1 -- Redacted_4700/LConn1 -- Redacted_3949/RConn1
  Redacted_9723/RConn1 -- Redacted_7804/RConn1
  Redacted_7804/LConn1 -- Redacted_2743/LConn1
  Redacted_9002/RConn1 -- Redacted_2743/RConn2
  Redacted_7804/LConn2 -- Redacted_1292/LConn1
  Redacted_7671/RConn1 -- Redacted_6636/LConn1
  Redacted_7671/LConn1 -- Redacted_1721/RConn1

== system Electrical_System_2018b_obfs/Redacted_1221/Redacted_7996/Redacted_7418/Redacted_4377/Redacted_6082/Redacted_144 ==
  Neutral_Negative : Subsystem  VariantControl=Variant1
  Positive_Neutral : Subsystem  VariantControl=Variant3
  Redacted_9503 : Subsystem  VariantControl=Variant2
  Redacted_3879 : PMIOPort  Side=Left
  Redacted_3368 : PMIOPort  Port=2  Side=Left
  Redacted_9451 : PMIOPort  Port=3  Side=Left
  Redacted_8432 : PMIOPort  Port=4  Side=Right
  Redacted_6806 : PMIOPort  Port=5  Side=Right

== system Electrical_System_2018b_obfs/Redacted_1221/Redacted_7996/Redacted_7418/Redacted_4377/Redacted_6082/Redacted_1502 ==
  Redacted_179 : fl_lib/Electrical/Electrical Elements/Switch  R_closed=tpfczkzopb Ohm  G_open=guejjlojqy 1/Ohm  Threshold=qftxyxgxji  i_specify=off  i_priority=None  i=fngbtljzex A  i_nominal_specify=off  i_nominal_unit=A  i_nominal_value=pjpooffzff  v_specify=off  v_priority=None  v=bhcpirmmxz V  v_nominal_specify=off  v_nominal_unit=V  v_nominal_value=jucxroftek
      settings: SourceProductName=Simscape
  Redacted_1815 : ee_lib/Semiconductors & Converters/Diode  ModelType=dqnklwqfci  Vf=xjiqjpnnfi V  Ron=irekdgqkjv Ohm  Goff=iqhtpofome S  prmExp=knojfylagq  I12=bqxijupuhm A  V12=vzuzujtkpl V  IS=ydgywotbys A  ec=ayrfemqefn  I1=delsjshmli A  V1=dnxxzmtubb V  RS=wmjpjwroih Ohm  Tmeas=qmtcdggbzc degC  N_series=hklouwtkux  N_parallel=jrdkdmsmgo  Rz=tovmqbbrol Ohm  BV=avdgidxjam V  C_param=glqkxeqcta  CJ=chsawhndir pF  CJ0=ayexifqzkz pF  VJ=zqcsdkhphs V  Mgrad=fkespxnvnl  Vvec=dqwhbiesyc V  Cvec=niiqpqslou pF  FC=cwbzovuqpz  Q_param=ylelzifboz  iRM=omgsmfewsp A  iF=ichmjhkctu A  didt=orrasyxhrt A/us  trr_factor=zdlyciflht  trr=twfpakhxfd ns  Qrr=ipntneuszo s*uA  TT=mwhbnzgoop ns  tau=pfrrcdfsln ns  T_param=ytujlpikwb  IS_T2=jerhvoexxa A  I1_T2=jvyzqlfhuc A  V1_T2=zarbmnbtma V  Tmeas2=vwndrphzjd degC  EG_param=pcxlgqdkwd  EG=vtwlzbuxst eV  XTI_param=jcpfqvyxtb  XTI=phmgnxxjxe  dBVdT=orxkvsgthq V/K  Tdevice=oqbwtmobso degC  i_specify=off  i_priority=None  i=yajbkzqnsh A  i_nominal_specify=off  i_nominal_unit=A  i_nominal_value=iwrztftqvf  v_specify=off  v_priority=None  v=ewtusmxpho V  v_nominal_specify=off  v_nominal_unit=V  v_nominal_value=syahoyjouu  i_capacitor_specify=off  i_capacitor_priority=None  i_capacitor=vxlszklfgf A  i_capacitor_nominal_specify=off  i_capacitor_nominal_unit=A  i_capacitor_nominal_value=duzmsfhmfv  v_capacitor_specify=off  v_capacitor_priority=None  v_capacitor=grvkfvfijd V  v_capacitor_nominal_specify=off  v_capacitor_nominal_unit=V  v_capacitor_nominal_value=zqixbhndtz  power_dissipated_specify=off  power_dissipated_priority=None  power_dissipated=bveezoguoz W  power_dissipated_nominal_specify=off  power_dissipated_nominal_unit=W  power_dissipated_nominal_value=wuvllpdufa  thermal_network_parameterization=rsoaylhfgu  Rth=owtikceqjs K/W  Rth_Foster=lmkblyjvxa K/W  thermal_mass_parameterization=edoczwbxzz  thermal_mass=ujhryaplvc J/K  thermal_mass_Foster=jnfsbuuslg J/K  thermal_time_constant=psujdozuva s  thermal_time_constant_Foster=kopgklxeqj s  thermal_mass_initial_temperatures=hdbyfhhyky degC
      settings: SourceProductName=Simscape Electrical  InternalSimscapePortConfiguration="{\"Bottom\":[],\"Left\":[{\"id\":\"p\",\"label\":\"\",\"type\":\"foundation.electrical.electrical\"},{\"id\":\"H\",\"label\":\"H\",\"type\":\"foundation.thermal.thermal\"}],\"Right\":[{\"id\":\"n\",\"label\":\"\",\"type\":\"foundation.electrical.electrical\"}],\"Top\":[]}"
  Redacted_309 : ee_lib/Passive/Thermal/Thermal Resistor  R=rlqpvmzzkw K/W  T_specify=off  T_priority=None  T=fayvhqopgz K  T_nominal_specify=off  T_nominal_unit=K  T_nominal_value=usakfhvqjr  Q_specify=off  Q_priority=None  Q=fradxufojf W  Q_nominal_specify=off  Q_nominal_unit=W  Q_nominal_value=vqlkwzshfu
      settings: SourceProductName=Simscape Electrical  SourceProductBaseCode=PS  InternalSimscapePortConfiguration="{\"Bottom\":[],\"Left\":[{\"id\":\"A\",\"label\":\"A\",\"type\":\"foundation.thermal.thermal\"}],\"Right\":[{\"id\":\"B\",\"label\":\"B\",\"type\":\"foundation.thermal.thermal\"}],\"Top\":[]}"
  Redacted_5427 : ee_lib/Semiconductors & Converters/Diode  ModelType=pvrilldlsl  Vf=exnaqxwczp V  Ron=byxhoupfbl Ohm  Goff=cclixdjcai S  prmExp=zgdvwqebkp  I12=aaaajndugd A  V12=zehnejyycd V  IS=bhumfyvqsp A  ec=qksjfmhjtn  I1=dzbxvwsdwy A  V1=qmphnapbom V  RS=ctsixmdfmz Ohm  Tmeas=voedtwdeem degC  N_series=zgsqwpgvsr  N_parallel=uokulxwqht  Rz=wfrfbwnojp Ohm  BV=qeyzssoejo V  C_param=svrqcrwtfc  CJ=dnwihzlyai pF  CJ0=qnrhvsekkn pF  VJ=qwvipkfmhu V  Mgrad=aiprwlrmva  Vvec=virrpuurya V  Cvec=inrcnfmckm pF  FC=vrvicjveyg  Q_param=uayuuepkqf  iRM=ktwoixrfbu A  iF=agmjhjxbxi A  didt=wopacoyifj A/us  trr_factor=mctfeqcgzf  trr=mcokfacpzx ns  Qrr=rvqtwqbvse s*uA  TT=wzilqodkkq ns  tau=ovarvjbymx ns  T_param=eagmvacwck  IS_T2=gceloirlpi A  I1_T2=cuojdhyufm A  V1_T2=ddoadsxlun V  Tmeas2=owwfcnzgyt degC  EG_param=htmtzkabpk  EG=znuuglnooo eV  XTI_param=rlgyybapxj  XTI=chmfxclcvd  dBVdT=mndckszxsr V/K  Tdevice=earqsgdndu degC  i_specify=off  i_priority=None  i=paejymtbgc A  i_nominal_specify=off  i_nominal_unit=A  i_nominal_value=ghormagyrn  v_specify=off  v_priority=None  v=mlxeomuyaz V  v_nominal_specify=off  v_nominal_unit=V  v_nominal_value=uzogtcjxmk  i_capacitor_specify=off  i_capacitor_priority=None  i_capacitor=reqkofmrwn A  i_capacitor_nominal_specify=off  i_capacitor_nominal_unit=A  i_capacitor_nominal_value=ofzxyeyrlg  v_capacitor_specify=off  v_capacitor_priority=None  v_capacitor=genvugjiwl V  v_capacitor_nominal_specify=off  v_capacitor_nominal_unit=V  v_capacitor_nominal_value=luaqihueqh  power_dissipated_specify=off  power_dissipated_priority=None  power_dissipated=xzkkuqjorb W  power_dissipated_nominal_specify=off  power_dissipated_nominal_unit=W  power_dissipated_nominal_value=gfhgakjqou  thermal_network_parameterization=kxvmefjoct  Rth=umlvscqlhx K/W  Rth_Foster=nlxizvbfxv K/W  thermal_mass_parameterization=yrswehzqhv  thermal_mass=uqwhhdrfmw J/K  thermal_mass_Foster=hjdthzjyej J/K  thermal_time_constant=fafhujuybb s  thermal_time_constant_Foster=rempkthvvv s  thermal_mass_initial_temperatures=zrogtrgfqe degC
      settings: SourceProductName=Simscape Electrical  InternalSimscapePortConfiguration="{\"Bottom\":[],\"Left\":[{\"id\":\"p\",\"label\":\"\",\"type\":\"foundation.electrical.electrical\"},{\"id\":\"H\",\"label\":\"H\",\"type\":\"foundation.thermal.thermal\"}],\"Right\":[{\"id\":\"n\",\"label\":\"\",\"type\":\"foundation.electrical.electrical\"}],\"Top\":[]}"
  Redacted_8072 : fl_lib/Electrical/Electrical Elements/Switch  R_closed=gnicoyhwdb Ohm  G_open=bwtrzzqkxe 1/Ohm  Threshold=btvjbsmnve  i_specify=off  i_priority=None  i=ffgvusnnup A  i_nominal_specify=off  i_nominal_unit=A  i_nominal_value=olaaofnvmv  v_specify=off  v_priority=None  v=hazqywjesu V  v_nominal_specify=off  v_nominal_unit=V  v_nominal_value=cujoeegpfv
      settings: SourceProductName=Simscape
  Redacted_8744 : ee_lib/Passive/Thermal/Thermal Resistor  R=qiiyhvuybo K/W  T_specify=off  T_priority=None  T=bmqsuewujl K  T_nominal_specify=off  T_nominal_unit=K  T_nominal_value=vyegnflrcg  Q_specify=off  Q_priority=None  Q=ozzgwrnnpp W  Q_nominal_specify=off  Q_nominal_unit=W  Q_nominal_value=zifsigreky
      settings: SourceProductName=Simscape Electrical  SourceProductBaseCode=PS  InternalSimscapePortConfiguration="{\"Bottom\":[],\"Left\":[{\"id\":\"A\",\"label\":\"A\",\"type\":\"foundation.thermal.thermal\"}],\"Right\":[{\"id\":\"B\",\"label\":\"B\",\"type\":\"foundation.thermal.thermal\"}],\"Top\":[]}"
  Redacted_9404 : ee_lib/Passive/Thermal/Thermal Resistor  R=vbnoxlgcgw K/W  T_specify=off  T_priority=None  T=umlukkevvv K  T_nominal_specify=off  T_nominal_unit=K  T_nominal_value=tnumztnkxu  Q_specify=off  Q_priority=None  Q=kisoetcdki W  Q_nominal_specify=off  Q_nominal_unit=W  Q_nominal_value=kojngerfgf
      settings: SourceProductName=Simscape Electrical  SourceProductBaseCode=PS  InternalSimscapePortConfiguration="{\"Bottom\":[],\"Left\":[{\"id\":\"A\",\"label\":\"A\",\"type\":\"foundation.thermal.thermal\"}],\"Right\":[{\"id\":\"B\",\"label\":\"B\",\"type\":\"foundation.thermal.thermal\"}],\"Top\":[]}"
  Redacted_6664 : PMIOPort  Side=Left
  Redacted_9877 : PMIOPort  Port=2  Side=Left
  Redacted_7484 : PMIOPort  Port=3  Side=Right
  Redacted_239 : PMIOPort  Port=4  Side=Right
  Redacted_1077 : PMIOPort  Port=5  Side=Left
  Redacted_1415 : PMIOPort  Port=6  Side=Right
  connections:
  Redacted_1815/LConn2 -- Redacted_309/LConn1
  Redacted_8744/RConn1 -- Redacted_1077/RConn1
  Redacted_239/RConn1 -- Redacted_179/RConn2
  Redacted_8072/RConn1 -- Redacted_179/RConn1 -- Redacted_1415/RConn1
  Redacted_9404/RConn1 -- Redacted_8744/LConn1 -- Redacted_309/RConn1
  Redacted_6664/RConn1 -- Redacted_5427/RConn1
  Redacted_5427/LConn1 -- Redacted_8072/LConn1
  Redacted_7484/RConn1 -- Redacted_8072/RConn2
  Redacted_5427/LConn2 -- Redacted_9404/LConn1
  Redacted_1815/RConn1 -- Redacted_179/LConn1
  Redacted_1815/LConn1 -- Redacted_9877/RConn1

== system Electrical_System_2018b_obfs/Redacted_1221/Redacted_7996/Redacted_7418/Redacted_4377/Redacted_6082/Redacted_1544 ==
  Neutral_Negative : Subsystem  VariantControl=Variant1
  Positive_Neutral : Subsystem  VariantControl=Variant3
  Redacted_4672 : Subsystem  VariantControl=Variant2
  Redacted_697 : PMIOPort  Side=Left
  Redacted_9789 : PMIOPort  Port=2  Side=Left
  Redacted_5820 : PMIOPort  Port=3  Side=Left
  Redacted_1167 : PMIOPort  Port=4  Side=Right
  Redacted_9408 : PMIOPort  Port=5  Side=Right
